simulink model "tp371876"  (Simulink 3.0)
settings: Solver=ode1  SolverMode=SingleTasking  StartTime=0.0  StopTime=inf  FixedStep=Ts  RelTol=1e-3
values from neighbouring files (symbols this model uses):
  K = 15    [uloha8.mat]
  Tfil = 2    [uloha8.mat]
  Ts = 0.5    [init_PI_arw_disc.m]    (also in init_step_resp1.m = 0.2; uloha7kvadra.mat = 0.1; uloha7linear.mat = 0.1; uloha8.mat = 0.2)
  Umax = 5    [init_PI_arw_disc.m]    (also in init_step_resp1.m; uloha7kvadra.mat; uloha7linear.mat; uloha8.mat)
  Umin = 0    [init_PI_arw_disc.m]    (also in init_step_resp1.m; uloha7kvadra.mat; uloha7linear.mat; uloha8.mat)
undefined symbols (not defined in the file or in its folder): T1
libraries: udaq28LT_lib x1
settings Model: LastModifiedBy=mato  ExtModeMexFile=rtwinext  ExtModeTrigDuration=100000  SaveFormat=Matrix  RTWSystemTargetFile=rtwin.tlc  RTWTemplateMakefile=rtwintmf  RTWOptions="-aCCOptimize=1 -aEnforceIntegerDowncast=1 -aExtMode=1 -aFoldNonRolledExpr=1 -aForceParamTrailComments=0 -aGenerateComments=1 -aGenerateReport=0 -aIncDataTypeInIds=0 -aIncHierarchyInIds=0 -aInlineInvariantSignals=0 -aInlinedPrmAccess=\"Literals\" -aLocalBlockOutputs=1 -aMaxRTWIdLen=31 -aPrefixModelToSubsysFcnNames=1 -aRTWVerbose=1 -aRebuildAll=1 -aRollThreshold=5 -aShowEliminatedStatements=1"

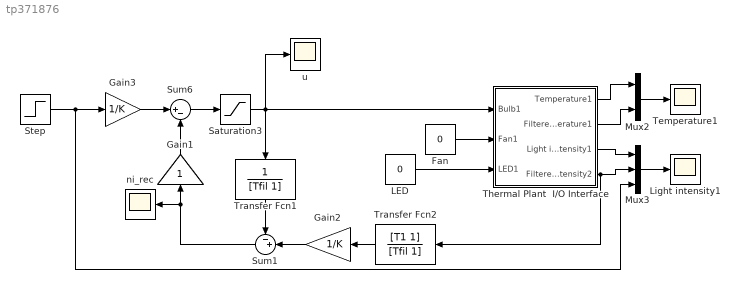
== system tp371876 ==
  Fan : Constant  Value=0
  Gain1 : Gain  Orientation=up  Gain=1  SaturateOnIntegerOverflow=on
  Gain2 : Gain  Orientation=left  Gain=1/K  SaturateOnIntegerOverflow=on
  Gain3 : Gain  Gain=1/K  SaturateOnIntegerOverflow=on
  LED : Constant  Value=0
  Light intensity1 : Scope
      settings: TickLabels=on  TimeRange=30  YMin=0  YMax=100  SaveName=yl  DataFormat=Matrix
  Mux2 : Mux  Inputs=2
  Mux3 : Mux  Inputs=3
  Saturation3 : Saturate  UpperLimit=Umax  LowerLimit=Umin
  Step : Step  Time=0  Before=0  After=25  SampleTime=Ts
  Sum1 : Sum  Orientation=left  Inputs=-+|  SaturateOnIntegerOverflow=on
  Sum6 : Sum  Inputs=|+-  SaturateOnIntegerOverflow=on
  Temperature1 : Scope
      settings: TickLabels=on  TimeRange=30  YMin=15  YMax=50  SaveName=yt  DataFormat=Matrix
  Thermal Plant  I/O Interface : Subsystem
      mask Display: disp('Thermo-optical\nPlant\nI/O Interface')
  Transfer Fcn1 : TransferFcn  Orientation=down  Numerator=[1 ]  Denominator=[Tfil 1]
  Transfer Fcn2 : TransferFcn  Orientation=left  Numerator=[T1 1]  Denominator=[Tfil 1]
  ni_rec : Scope
      settings: TimeRange=auto  YMin=1.5  YMax=2.7  SaveName=ni_rec  DataFormat=Matrix  Decimation=10  SampleInput=on  SampleTime=Ts
  u : Scope
      settings: TimeRange=100  YMin=-0.5  YMax=5.5  SaveName=u  DataFormat=Matrix  Decimation=10  SampleInput=on  SampleTime=Ts
  wires:
  Transfer Fcn1/1 -> Sum1/1
  Sum1/1 -> ni_rec/1, Gain1/1
  Gain1/1 -> Sum6/2
  Transfer Fcn2/1 -> Gain2/1
  Gain2/1 -> Sum1/2
  Sum6/1 -> Saturation3/1
  Saturation3/1 -> u/1, Transfer Fcn1/1, Thermal Plant  I/O Interface/1(Bulb1)
  Gain3/1 -> Sum6/1
  Step/1 -> Gain3/1, Mux3/3
  Mux2/1 -> Temperature1/1
  Mux3/1 -> Light intensity1/1
  Fan/1 -> Thermal Plant  I/O Interface/2(Fan1)
  LED/1 -> Thermal Plant  I/O Interface/3(LED1)
  Thermal Plant  I/O Interface/1(Temperature1) -> Mux2/1
  Thermal Plant  I/O Interface/2(Filtered  temperature1) -> Mux2/2
  Thermal Plant  I/O Interface/3(Light intensity1) -> Mux3/1
  Thermal Plant  I/O Interface/4(Filtered  light intensity2) -> Mux3/2, Transfer Fcn2/1

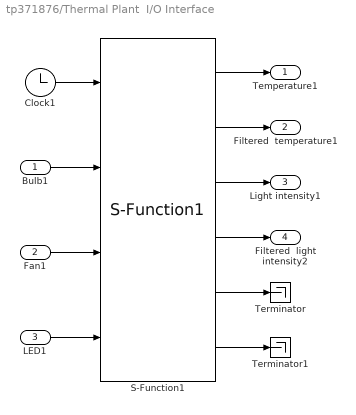
== system tp371876/Thermal Plant  I/O Interface ==
  Bulb1 : Inport  Port=1  PortWidth=-1  SampleTime=-1  DataType=auto
      settings: SignalType=auto
  Fan1 : Inport  Port=2  PortWidth=-1  SampleTime=-1  DataType=auto
      settings: SignalType=auto
  LED1 : Inport  Port=3  PortWidth=-1  SampleTime=-1  DataType=auto
      settings: SignalType=auto
  Clock1 : Clock
      settings: DisplayTime=off  Decimation=10
  S-Function1 : udaq28LT_lib/S-Function1  Priority=1  com_port=COM3  Ts=Ts  events_ot=2  rd_timeout=Ts/2*1000  matlab_prior=ABOVE_NORMAL_PRIORITY  warning=on  printout=off
  Terminator : Terminator
  Terminator1 : Terminator
  Temperature1 : Outport  Port=1
  Filtered  temperature1 : Outport  Port=2
  Light intensity1 : Outport  Port=3
  Filtered  light intensity2 : Outport  Port=4
  wires:
  S-Function1/1 -> Temperature1/1
  S-Function1/2 -> Filtered  temperature1/1
  Clock1/1 -> S-Function1/1
  Bulb1/1 -> S-Function1/2
  Fan1/1 -> S-Function1/3
  S-Function1/3 -> Light intensity1/1
  S-Function1/4 -> Filtered  light intensity2/1
  S-Function1/5 -> Terminator/1
  S-Function1/6 -> Terminator1/1
  LED1/1 -> S-Function1/4
